simulink model "control_balance"  (R2017a)
settings: Solver=VariableStepAuto  StartTime=0.0  StopTime=10.0  RelTol=1e-3
values from neighbouring files (symbols this model uses):
  sample_period_Ts = 0.08    [setup.m]
undefined symbols (not defined in the file or in its folder): phi_u_z_den, phi_u_z_num
libraries: simulink x1
settings Model: Creator=Horia  LastModifiedBy=Horia

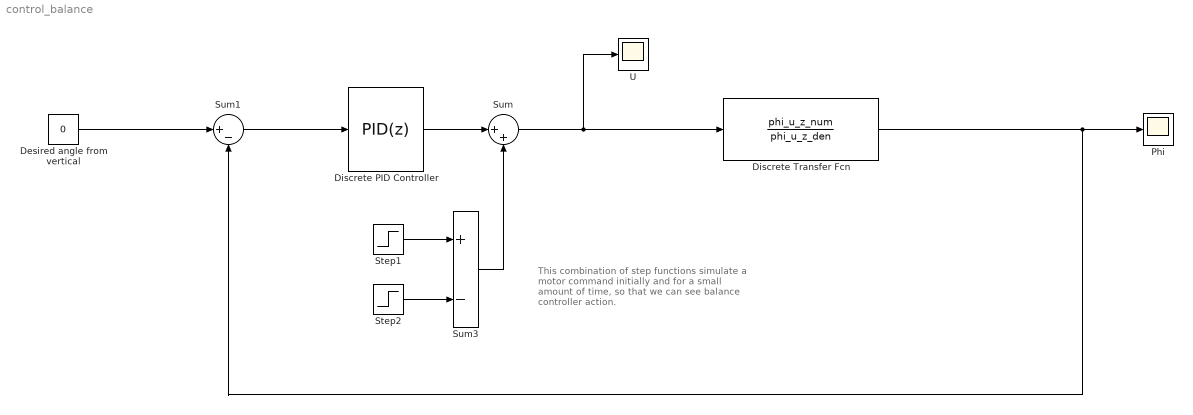
== system control_balance ==
  note: This combination of step functions simulate
      | a motor command initially and for a small
      | amount of time, so that we can see
      | balance controller action.
  Desired angle from vertical : Constant  Value=0
  Discrete Transfer Fcn : DiscreteTransferFcn  Numerator=phi_u_z_num  Denominator=phi_u_z_den  SampleTime=sample_period_Ts
  Discrete PID Controller : simulink/Continuous/PID Controller  Controller=PID  TimeDomain=Discrete-time  SampleTime=-1  IntegratorMethod=Forward Euler  FilterMethod=Forward Euler  Form=Parallel  UseFilter=on  ControllerParametersSource=internal  P=9.44930273653691  I=14.3277103307661  D=1.28333432861171  N=24.2402296183356  InitialConditionSource=internal  InitialConditionForIntegrator=0  InitialConditionForFilter=0  ExternalReset=none  LimitOutput=off  UpperSaturationLimit=inf  LowerSaturationLimit=-inf  LinearizeAsGain=off  AntiWindupMode=none  Kb=1  TrackingMode=off  Kt=1  PParamMin=[]  PParamMax=[]  IParamMin=[]  IParamMax=[]  DParamMin=[]  DParamMax=[]  NParamMin=[]  NParamMax=[]  KbParamMin=[]  KbParamMax=[]  KtParamMin=[]  KtParamMax=[]  POutMin=[]  POutMax=[]  IOutMin=[]  IOutMax=[]  DOutMin=[]  DOutMax=[]  NOutMin=[]  NOutMax=[]  KbOutMin=[]  KbOutMax=[]  KtOutMin=[]  KtOutMax=[]  IntegratorOutMin=[]  IntegratorOutMax=[]  FilterOutMin=[]  FilterOutMax=[]  SumOutMin=[]  SumOutMax=[]  SumI1OutMin=[]  SumI1OutMax=[]  SumI2OutMin=[]  SumI2OutMax=[]  SumI3OutMin=[]  SumI3OutMax=[]  SumDOutMin=[]  SumDOutMax=[]  SaturationOutMin=[]  SaturationOutMax=[]  IntegratorContinuousStateAttributes=''  IntegratorStateMustResolveToSignalObject=off  IntegratorRTWStateStorageClass=Auto  FilterContinuousStateAttributes=''  FilterStateMustResolveToSignalObject=off  FilterRTWStateStorageClass=Auto  DifferentiatorICPrevScaledInput=0  DifferentiatorOutMin=[]  DifferentiatorOutMax=[]  InitialConditionSetting=State (most efficient)
  Phi : Scope
  Step1 : Step  After=2  SampleTime=0
  Step2 : Step  Time=1.1  After=2  SampleTime=0
  Sum : Sum  Inputs=|++
  Sum1 : Sum  Inputs=|+-
  Sum3 : Sum  Inputs=+-
  U : Scope
  wires:
  Sum3/1 -> Sum/2
  Step1/1 -> Sum3/1
  Discrete PID Controller/1 -> Sum/1
  Desired angle from vertical/1 -> Sum1/1
  Sum1/1 -> Discrete PID Controller/1
  Sum/1 -> Discrete Transfer Fcn/1, U/1
  Step2/1 -> Sum3/2
  Discrete Transfer Fcn/1 -> Sum1/2, Phi/1
